simulink library "component_lib"  (R2023a)
settings: Solver=VariableStepAuto  StartTime=0.0  StopTime=10.0  RelTol=1e-3
undefined symbols (not defined in the file or in its folder): ECCV_r, par, R1234yf_ph, V_nom
libraries: base_lib x258, $bdroot x212, simulink x2, slpidlib x1
(part 4 of 7)

== system component_lib/Fuel Cell System/Subsystem1 ==
  note: Rolling Fuel Consumption Calculation [kg/100km]
  In1 : Inport
  Add1 : Sum
  Constant6 : Constant
  Constant7 : Constant  Value=100e3
  Demux : Demux
  Divide : Product  Inputs=**/
  Gain1 : Gain  Gain=-1
  Integrator : Integrator
  SC0002_signalRead11 : $bdroot/Data & Control/SC0002_signalRead  SigName=fuelConsumption
  SC0002_signalRead5 : $bdroot/Data & Control/SC0002_signalRead  SigName=hydrogenFlow
  SC0003_signalWrite1 : $bdroot/Data & Control/SC0003_signalWrite  SigName=distance
  Terminator : Terminator
  Terminator1 : Terminator
  Terminator2 : Terminator
  wires:
  Integrator/1 -> Divide/1
  Constant7/1 -> Divide/2
  SC0003_signalWrite1/1 -> Add1/1
  Demux/1 -> Gain1/1
  Add1/1 -> Divide/3
  Constant6/1 -> Add1/2
  Divide/1 -> SC0002_signalRead11/1
  Gain1/1 -> SC0002_signalRead5/1, Integrator/1
  In1/1 -> Demux/1
  Demux/3 -> Terminator1/1
  Demux/4 -> Terminator2/1
  Demux/2 -> Terminator/1

== system component_lib/Gas Exchange/GE0001_humidGasSupply ==
  Constant : Constant  Value=par.p_tot
  Constant1 : Constant  Value=par.RH
  Constant2 : Constant  Value=par.T
  Constant3 : Constant  Value=par.x_H2
  Constant4 : Constant  Value=par.x_O2
  F0010_pressureSupply.m : base_lib/F0010_gasFlow/F0010_pressureSupply.m  SystemSampleTime=-1  VariantActivationTime=update diagram  Latency=0  AutoFrameSizeCalculation=off
  F0010_vaporSaturationPressure.m : base_lib/F0010_gasFlow/F0010_vaporSaturationPressure.m  SystemSampleTime=-1  VariantActivationTime=update diagram  Latency=0  AutoFrameSizeCalculation=off
  p (p x 4) : Outport
  T [K] : Outport  Port=2
  wires:
  Constant2/1 -> T [K]/1, F0010_vaporSaturationPressure.m/1
  Constant/1 -> F0010_pressureSupply.m/1
  F0010_vaporSaturationPressure.m/1 -> F0010_pressureSupply.m/5
  Constant1/1 -> F0010_pressureSupply.m/4
  Constant3/1 -> F0010_pressureSupply.m/2
  Constant4/1 -> F0010_pressureSupply.m/3
  F0010_pressureSupply.m/1 -> p (p x 4)/1

== system component_lib/Gas Exchange/GE0002_dynHumidGasSupply ==
  T [K] : Inport
  p_ref [Pa] : Inport  Port=2
  RH [-] : Inport  Port=3
  Constant : Constant  Value=x_H2_dry
  Constant1 : Constant  Value=x_O2_dry
  F0010_pressureSupply.m : base_lib/F0010_gasFlow/F0010_pressureSupply.m  SystemSampleTime=-1  VariantActivationTime=update diagram  Latency=0  AutoFrameSizeCalculation=off
  F0010_vaporSaturationPressure.m : base_lib/F0010_gasFlow/F0010_vaporSaturationPressure.m  SystemSampleTime=-1  VariantActivationTime=update diagram  Latency=0  AutoFrameSizeCalculation=off
  p (p x 4) : Outport
  T_out [K] : Outport  Port=2
  wires:
  p_ref [Pa]/1 -> F0010_pressureSupply.m/1
  T [K]/1 -> F0010_vaporSaturationPressure.m/1, T_out [K]/1
  F0010_vaporSaturationPressure.m/1 -> F0010_pressureSupply.m/5
  RH [-]/1 -> F0010_pressureSupply.m/4
  F0010_pressureSupply.m/1 -> p (p x 4)/1
  Constant/1 -> F0010_pressureSupply.m/2
  Constant1/1 -> F0010_pressureSupply.m/3

== system component_lib/Gas Exchange/GE0007_hydrogenTank ==
  W_H2 [kg/s] : Inport
  Actuator dynamics : TransferFcn  Denominator=[0.1 1]
  Constant : Constant  Value=0
  Constant2 : Constant  Value=par.V
  Constant3 : Constant  Value=par.T_tank
  Constant4 : Constant  Value=0
  Constant5 : Constant  Value=par.m0
  Constant6 : Constant  Value=par.m0
  Constant7 : Constant  Value=par.M_j(1)
  Constant8 : Constant  Value=par.init_SOC
  Constant9 : Constant  Value=0
  Divide{,1..2,4} (4 alike) : Product  Inputs=*/
  F0005_enthalpy.m : base_lib/F0005_h2Thermodynamics/F0005_enthalpy.m  SystemSampleTime=-1  VariantActivationTime=update diagram  Latency=0  AutoFrameSizeCalculation=off
  F0005_pressure.m : base_lib/F0005_h2Thermodynamics/F0005_pressure.m  SystemSampleTime=-1  VariantActivationTime=update diagram  Latency=0  AutoFrameSizeCalculation=off
  Gain : Gain  Gain=-1
  Hydrogen ideal gas molar specific heat : Constant  Value=par.cp_j(1) .* par.M_j(1);
  Integrator Limited : Integrator  InitialConditionSource=external  LimitOutput=on  LowerSaturationLimit=0
  Mux : Mux
  Product : Product
  Standard state molar enthalpy : Constant  Value=par.h0
  Sum : Sum  Inputs=|+-
  Sum1 : Sum  Inputs=|++
  standard state temperature : Constant  Value=par.T0
  W [kg/s] : Outport
  T [K] : Outport  Port=2
  SOC [-] : Outport  Port=3
  p _tank [Pa] : Outport  Port=4
  wires:
  Integrator Limited/1 -> Divide1/1, Divide2/1
  Constant2/1 -> Divide1/2
  Constant3/1 -> F0005_pressure.m/1, F0005_enthalpy.m/1
  F0005_pressure.m/1 -> p _tank [Pa]/1
  Divide2/1 -> SOC [-]/1
  Hydrogen ideal gas molar specific heat/1 -> Divide/2
  Divide1/1 -> Divide4/1
  Constant7/1 -> Divide4/2
  Divide4/1 -> F0005_enthalpy.m/2, F0005_pressure.m/2
  F0005_enthalpy.m/1 -> Sum/1
  Standard state molar enthalpy/1 -> Sum/2
  Sum/1 -> Divide/1
  Divide/1 -> Sum1/1
  standard state temperature/1 -> Sum1/2
  Sum1/1 -> T [K]/1
  Constant5/1 -> Divide2/2
  Constant6/1 -> Product/1
  Product/1 -> Integrator Limited/2
  Constant8/1 -> Product/2
  Constant9/1 -> Mux/4
  Constant/1 -> Mux/2
  Constant4/1 -> Mux/3
  Actuator dynamics/1 -> Gain/1, Mux/1
  Mux/1 -> W [kg/s]/1
  Gain/1 -> Integrator Limited/1
  W_H2 [kg/s]/1 -> Actuator dynamics/1

== system component_lib/Gas Exchange/GE0008_gasProperties ==
  p (p x 4) : Inport
  T [K] : Inport  Port=2
  Demux : Demux
  Divide : Product  Inputs=*/
  F0010_vaporSaturationPressure.m : base_lib/F0010_gasFlow/F0010_vaporSaturationPressure.m  SystemSampleTime=-1  VariantActivationTime=update diagram  Latency=0  AutoFrameSizeCalculation=off
  Mux : Mux
  Sum : Sum  Inputs=|+|
  p [Pa] : Outport
  RH [-] : Outport  Port=2
  wires:
  Sum/1 -> p [Pa]/1
  p (p x 4)/1 -> Demux/1
  Demux/1 -> Mux/1
  Demux/2 -> Mux/2
  Demux/3 -> Divide/1, Mux/3
  Demux/4 -> Mux/4
  Mux/1 -> Sum/1
  Divide/1 -> RH [-]/1
  F0010_vaporSaturationPressure.m/1 -> Divide/2
  T [K]/1 -> F0010_vaporSaturationPressure.m/1

== system component_lib/Gas Exchange/GE0009_controlVolume ==
  note: Pressure
  note: Mass flow contribution
      | to pressure dynamics
  dW [kg/s x 4] : Inport
  T [K] : Inport  Port=2
  Constant : Constant  Value=par.p0
  Constant1 : Constant  Value=par.RH0
  Constant3 : Constant  Value=par.V
  Constant5 : Constant  Value=par.x0_H2
  Constant6 : Constant  Value=par.x0_O2
  Divide1 : Product  Inputs=***/
  F0010_pressureSupply.m : base_lib/F0010_gasFlow/F0010_pressureSupply.m  SystemSampleTime=-1  VariantActivationTime=update diagram  Latency=0  AutoFrameSizeCalculation=off
      settings: LibrarySourceBlock=|
      | simulink/User-Defined
      | Functions/MATLAB Function
  F0010_vaporSaturationPressure.m : base_lib/F0010_gasFlow/F0010_vaporSaturationPressure.m  SystemSampleTime=-1  VariantActivationTime=update diagram  Latency=0  AutoFrameSizeCalculation=off
      settings: LibrarySourceBlock=|
      | simulink/User-Defined
      | Functions/MATLAB Function
  Gas constants : Constant  Value=par.R_j
  Integrator Limited1 : Integrator  InitialConditionSource=external  LimitOutput=on  LowerSaturationLimit=0
  p [Pa x 4] : Outport
  wires:
  Integrator Limited1/1 -> p [Pa x 4]/1
  Constant/1 -> F0010_pressureSupply.m/1
  F0010_pressureSupply.m/1 -> Integrator Limited1/2
  dW [kg/s x 4]/1 -> Divide1/1
  Divide1/1 -> Integrator Limited1/1
  Constant3/1 -> Divide1/4
  Gas constants/1 -> Divide1/2
  F0010_vaporSaturationPressure.m/1 -> F0010_pressureSupply.m/5
  Constant1/1 -> F0010_pressureSupply.m/4
  Constant5/1 -> F0010_pressureSupply.m/2
  Constant6/1 -> F0010_pressureSupply.m/3
  T [K]/1 -> F0010_vaporSaturationPressure.m/1, Divide1/3

== system component_lib/Gas Exchange/GE0010_compressibleRestriction ==
  p_us [Pa x 4] : Inport
  T_us [K] : Inport  Port=2
  p_ds [Pa x 4] : Inport  Port=3
  Area : Constant  Value=pi*(D_t/2)^2
  F0010_compressibleRestriction.m : base_lib/F0010_gasFlow/F0010_compressibleRestriction.m  SystemSampleTime=-1  VariantActivationTime=update diagram  Latency=0  AutoFrameSizeCalculation=off
      settings: LibrarySourceBlock=|
      | simulink/User-Defined
      | Functions/MATLAB Function
  F0010_mixtureProperties.m : base_lib/F0010_gasFlow/F0010_mixtureProperties.m  SystemSampleTime=-1  VariantActivationTime=update diagram  Latency=0  AutoFrameSizeCalculation=off
      settings: LibrarySourceBlock=|
      | simulink/User-Defined
      | Functions/MATLAB Function
  F0010_multicomponentFlow.m : base_lib/F0010_gasFlow/F0010_multicomponentFlow.m  SystemSampleTime=-1  VariantActivationTime=update diagram  Latency=0  AutoFrameSizeCalculation=off
      settings: LibrarySourceBlock=|
      | simulink/User-Defined
      | Functions/MATLAB Function
  Sum : Sum  Inputs=+
  Sum1 : Sum  Inputs=+
  Terminator : Terminator
  Terminator1 : Terminator
  W [kg/s x 4] : Outport
  T_ds [K] : Outport  Port=2
  wires:
  T_us [K]/1 -> F0010_compressibleRestriction.m/3, T_ds [K]/1
  p_us [Pa x 4]/1 -> Sum/1, F0010_mixtureProperties.m/1, F0010_multicomponentFlow.m/1
  p_ds [Pa x 4]/1 -> Sum1/1
  Sum/1 -> F0010_compressibleRestriction.m/1
  Sum1/1 -> F0010_compressibleRestriction.m/2
  F0010_compressibleRestriction.m/1 -> F0010_multicomponentFlow.m/2
  F0010_multicomponentFlow.m/1 -> W [kg/s x 4]/1
  F0010_mixtureProperties.m/2 -> F0010_compressibleRestriction.m/4
  F0010_mixtureProperties.m/4 -> F0010_compressibleRestriction.m/5
  F0010_mixtureProperties.m/1 -> Terminator/1
  F0010_mixtureProperties.m/3 -> Terminator1/1
  Area/1 -> F0010_compressibleRestriction.m/6

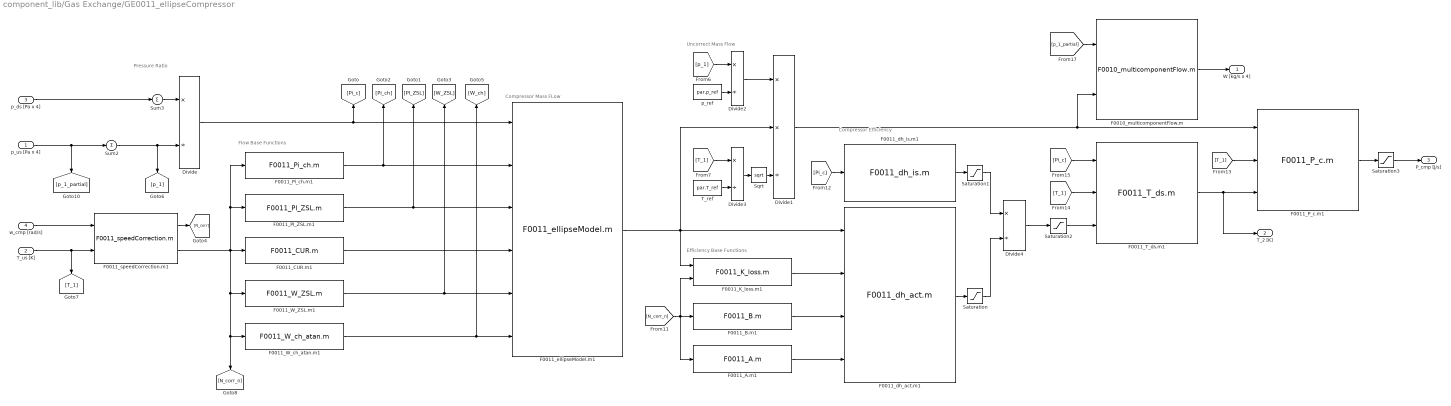
== system component_lib/Gas Exchange/GE0011_ellipseCompressor ==
  note: Compressor Mass FLow
  note: Compressor Efficiency
  note: Efficiency Base Functions
  note: Pressure Ratio
  note: Flow Base Functions
  note: Uncorrect Mass Flow
  p_us [Pa x 4] : Inport
  T_us [K] : Inport  Port=2
  p_ds [Pa x 4] : Inport  Port=3
  w_cmp [rad/s] : Inport  Port=4
  Divide{,2..4} (4 alike) : Product  Inputs=*/
  Divide1 : Product  Inputs=**/
  F0010_multicomponentFlow.m : base_lib/F0010_gasFlow/F0010_multicomponentFlow.m  SystemSampleTime=-1  VariantActivationTime=update diagram  Latency=0  AutoFrameSizeCalculation=off
      settings: LibrarySourceBlock=|
      | simulink/User-Defined
      | Functions/MATLAB Function
  F0011_A.m1 : base_lib/F0011_ellipseCompressor/F0011_A.m  SystemSampleTime=-1  VariantActivationTime=update diagram  Latency=0  AutoFrameSizeCalculation=off
      settings: LibrarySourceBlock=|
      | simulink/User-Defined
      | Functions/MATLAB Function
  F0011_B.m1 : base_lib/F0011_ellipseCompressor/F0011_B.m  SystemSampleTime=-1  VariantActivationTime=update diagram  Latency=0  AutoFrameSizeCalculation=off
      settings: LibrarySourceBlock=|
      | simulink/User-Defined
      | Functions/MATLAB Function
  F0011_CUR.m1 : base_lib/F0011_ellipseCompressor/F0011_CUR.m  SystemSampleTime=-1  VariantActivationTime=update diagram  Latency=0  AutoFrameSizeCalculation=off
      settings: LibrarySourceBlock=|
      | simulink/User-Defined
      | Functions/MATLAB Function
  F0011_K_loss.m1 : base_lib/F0011_ellipseCompressor/F0011_K_loss.m  SystemSampleTime=-1  VariantActivationTime=update diagram  Latency=0  AutoFrameSizeCalculation=off
      settings: LibrarySourceBlock=|
      | simulink/User-Defined
      | Functions/MATLAB Function
  F0011_PI_ZSL.m1 : base_lib/F0011_ellipseCompressor/F0011_PI_ZSL.m  SystemSampleTime=-1  VariantActivationTime=update diagram  Latency=0  AutoFrameSizeCalculation=off
      settings: LibrarySourceBlock=|
      | simulink/User-Defined
      | Functions/MATLAB Function
  F0011_P_c.m1 : base_lib/F0011_ellipseCompressor/F0011_P_c.m  SystemSampleTime=-1  VariantActivationTime=update diagram  Latency=0  AutoFrameSizeCalculation=off
      settings: LibrarySourceBlock=|
      | simulink/User-Defined
      | Functions/MATLAB Function
  F0011_Pi_ch.m1 : base_lib/F0011_ellipseCompressor/F0011_Pi_ch.m  SystemSampleTime=-1  VariantActivationTime=update diagram  Latency=0  AutoFrameSizeCalculation=off
      settings: LibrarySourceBlock=|
      | simulink/User-Defined
      | Functions/MATLAB Function
  F0011_T_ds.m1 : base_lib/F0011_ellipseCompressor/F0011_T_ds.m  SystemSampleTime=-1  VariantActivationTime=update diagram  Latency=0  AutoFrameSizeCalculation=off
      settings: LibrarySourceBlock=|
      | simulink/User-Defined
      | Functions/MATLAB Function
  F0011_W_ZSL.m1 : base_lib/F0011_ellipseCompressor/F0011_W_ZSL.m  SystemSampleTime=-1  VariantActivationTime=update diagram  Latency=0  AutoFrameSizeCalculation=off
      settings: LibrarySourceBlock=|
      | simulink/User-Defined
      | Functions/MATLAB Function
  F0011_W_ch_atan.m1 : base_lib/F0011_ellipseCompressor/F0011_W_ch_atan.m  SystemSampleTime=-1  VariantActivationTime=update diagram  Latency=0  AutoFrameSizeCalculation=off
      settings: LibrarySourceBlock=|
      | simulink/User-Defined
      | Functions/MATLAB Function
  F0011_dh_act.m1 : base_lib/F0011_ellipseCompressor/F0011_dh_act.m  SystemSampleTime=-1  VariantActivationTime=update diagram  Latency=0  AutoFrameSizeCalculation=off
      settings: LibrarySourceBlock=|
      | simulink/User-Defined
      | Functions/MATLAB Function
  F0011_dh_is.m1 : base_lib/F0011_ellipseCompressor/F0011_dh_is.m  SystemSampleTime=-1  VariantActivationTime=update diagram  Latency=0  AutoFrameSizeCalculation=off
      settings: LibrarySourceBlock=|
      | simulink/User-Defined
      | Functions/MATLAB Function
  F0011_ellipseModel.m1 : base_lib/F0011_ellipseCompressor/F0011_ellipseModel.m  SystemSampleTime=-1  VariantActivationTime=update diagram  Latency=0  AutoFrameSizeCalculation=off
      settings: LibrarySourceBlock=|
      | simulink/User-Defined
      | Functions/MATLAB Function
  F0011_speedCorrection.m1 : base_lib/F0011_ellipseCompressor/F0011_speedCorrection.m  SystemSampleTime=-1  VariantActivationTime=update diagram  Latency=0  AutoFrameSizeCalculation=off
      settings: LibrarySourceBlock=|
      | simulink/User-Defined
      | Functions/MATLAB Function
  Saturation : Saturate  UpperLimit=inf  LowerLimit=1e-4
  Saturation1 : Saturate  UpperLimit=inf  LowerLimit=1e-4
  Saturation2 : Saturate  UpperLimit=1  LowerLimit=1e-3
  Saturation3 : Saturate  UpperLimit=inf  LowerLimit=0
  Sqrt : Sqrt
  Sum2 : Sum  Inputs=|+|
  Sum3 : Sum  Inputs=|+|
  T_ref : Constant  Value=par.T_ref
  p_ref : Constant  Value=par.p_ref
  W [kg/s x 4] : Outport
  T_2 [K] : Outport  Port=2
  P_cmp [J/s] : Outport  Port=3
  wires:
  Sum3/1 -> Divide/1
  T_us [K]/1 -> F0011_speedCorrection.m1/2, [T_1]
  F0011_CUR.m1/1 -> F0011_ellipseModel.m1/4
  F0011_PI_ZSL.m1/1 -> F0011_ellipseModel.m1/3, [PI_ZSL]
  F0011_W_ZSL.m1/1 -> F0011_ellipseModel.m1/5, [W_ZSL]
  F0011_W_ch_atan.m1/1 -> F0011_ellipseModel.m1/6, [W_ch]
  F0011_speedCorrection.m1/2 -> F0011_CUR.m1/1, F0011_W_ZSL.m1/1, F0011_W_ch_atan.m1/1, [N_corr_n], F0011_PI_ZSL.m1/1, F0011_Pi_ch.m1/1
  Divide/1 -> F0011_ellipseModel.m1/1, [Pi_c]
  F0011_speedCorrection.m1/1 -> [N_corr]
  Divide1/1 -> F0011_P_c.m1/1, F0010_multicomponentFlow.m/2
  p_ref/1 -> Divide2/2
  Divide2/1 -> Divide1/1
  [p_1] -> Divide2/1
  [T_1] -> Divide3/1
  T_ref/1 -> Divide3/2
  Divide3/1 -> Sqrt/1
  Sqrt/1 -> Divide1/3
  F0011_Pi_ch.m1/1 -> F0011_ellipseModel.m1/2, [Pi_ch]
  F0011_K_loss.m1/1 -> F0011_dh_act.m1/2
  F0011_B.m1/1 -> F0011_dh_act.m1/3
  F0011_A.m1/1 -> F0011_dh_act.m1/4
  [N_corr_n] -> F0011_A.m1/1, F0011_B.m1/1, F0011_K_loss.m1/2
  [Pi_c] -> F0011_dh_is.m1/1
  F0011_dh_act.m1/1 -> Saturation/1
  F0011_dh_is.m1/1 -> Saturation1/1
  Saturation1/1 -> Divide4/1
  Saturation/1 -> Divide4/2
  Divide4/1 -> Saturation2/1
  Saturation2/1 -> F0011_T_ds.m1/3
  F0011_T_ds.m1/1 -> F0011_P_c.m1/3, T_2 [K]/1
  [T_1] -> F0011_P_c.m1/2
  [T_1] -> F0011_T_ds.m1/2
  [Pi_c] -> F0011_T_ds.m1/1
  w_cmp [rad/s]/1 -> F0011_speedCorrection.m1/1
  p_us [Pa x 4]/1 -> Sum2/1, [p_1_partial]
  Sum2/1 -> Divide/2, [p_1]
  [p_1_partial] -> F0010_multicomponentFlow.m/1
  F0010_multicomponentFlow.m/1 -> W [kg/s x 4]/1
  F0011_ellipseModel.m1/1 -> F0011_dh_act.m1/1, F0011_K_loss.m1/1, Divide1/2
  p_ds [Pa x 4]/1 -> Sum3/1
  F0011_P_c.m1/1 -> Saturation3/1
  Saturation3/1 -> P_cmp [J/s]/1

== system component_lib/Gas Exchange/GE0012_throttle ==
  p_us [Pa x 4] : Inport
  T_us [K] : Inport  Port=2
  p_ds [Pa x 4] : Inport  Port=3
  alpha [-] : Inport  Port=4
  F0010_compressibleRestriction.m : base_lib/F0010_gasFlow/F0010_compressibleRestriction.m  SystemSampleTime=-1  VariantActivationTime=update diagram  Latency=0  AutoFrameSizeCalculation=off
      settings: LibrarySourceBlock=|
      | simulink/User-Defined
      | Functions/MATLAB Function
  F0010_mixtureProperties.m : base_lib/F0010_gasFlow/F0010_mixtureProperties.m  SystemSampleTime=-1  VariantActivationTime=update diagram  Latency=0  AutoFrameSizeCalculation=off
      settings: LibrarySourceBlock=|
      | simulink/User-Defined
      | Functions/MATLAB Function
  F0010_multicomponentFlow.m : base_lib/F0010_gasFlow/F0010_multicomponentFlow.m  SystemSampleTime=-1  VariantActivationTime=update diagram  Latency=0  AutoFrameSizeCalculation=off
      settings: LibrarySourceBlock=|
      | simulink/User-Defined
      | Functions/MATLAB Function
  F0010_throttleArea.m : base_lib/F0010_gasFlow/F0010_throttleArea.m  SystemSampleTime=-1  VariantActivationTime=update diagram  Latency=0  AutoFrameSizeCalculation=off
      settings: LibrarySourceBlock=|
      | simulink/User-Defined
      | Functions/MATLAB Function
  Sum : Sum  Inputs=+
  Sum1 : Sum  Inputs=+
  Terminator : Terminator
  Terminator1 : Terminator
  W [kg/s x 4] : Outport
  T_out [K] : Outport  Port=2
  wires:
  T_us [K]/1 -> F0010_compressibleRestriction.m/3, T_out [K]/1
  p_us [Pa x 4]/1 -> Sum/1, F0010_mixtureProperties.m/1, F0010_multicomponentFlow.m/1
  p_ds [Pa x 4]/1 -> Sum1/1
  Sum/1 -> F0010_compressibleRestriction.m/1
  Sum1/1 -> F0010_compressibleRestriction.m/2
  F0010_compressibleRestriction.m/1 -> F0010_multicomponentFlow.m/2
  F0010_multicomponentFlow.m/1 -> W [kg/s x 4]/1
  F0010_mixtureProperties.m/2 -> F0010_compressibleRestriction.m/4
  F0010_mixtureProperties.m/4 -> F0010_compressibleRestriction.m/5
  F0010_mixtureProperties.m/1 -> Terminator/1
  F0010_mixtureProperties.m/3 -> Terminator1/1
  F0010_throttleArea.m/1 -> F0010_compressibleRestriction.m/6
  alpha [-]/1 -> F0010_throttleArea.m/1

== system component_lib/Gas Exchange/GE0013_ejector ==
  p_p [Pa x 4] : Inport
  T_p [K] : Inport  Port=2
  p_s [Pa x 4] : Inport  Port=3
  T_s [K] : Inport  Port=4
  p_b [Pa x 4] : Inport  Port=5
  Divide : Product  Inputs=*/
  F0010_ejectorModel.m : base_lib/F0010_gasFlow/F0010_ejectorModel.m  SystemSampleTime=-1  VariantActivationTime=update diagram  Latency=0  AutoFrameSizeCalculation=off
      settings: LibrarySourceBlock=|
      | simulink/User-Defined
      | Functions/MATLAB Function
  F0010_multicomponentFlow.m : base_lib/F0010_gasFlow/F0010_multicomponentFlow.m  SystemSampleTime=-1  VariantActivationTime=update diagram  Latency=0  AutoFrameSizeCalculation=off
  F0010_multicomponentFlow.m1 : base_lib/F0010_gasFlow/F0010_multicomponentFlow.m  SystemSampleTime=-1  VariantActivationTime=update diagram  Latency=0  AutoFrameSizeCalculation=off
  F0010_vaporSaturationPressure.m : base_lib/F0010_gasFlow/F0010_vaporSaturationPressure.m  SystemSampleTime=-1  VariantActivationTime=update diagram  Latency=0  AutoFrameSizeCalculation=off
  Selector : Selector  InputPortWidth=4  IndexOptions=Index vector (dialog)  Indices=3  OutputSizes=1
  Sum : Sum  Inputs=+
  Sum1 : Sum  Inputs=+
  Sum2 : Sum  Inputs=+
  W_p [kg/s] : Outport
  W_s [kg/s] : Outport  Port=2
  phi [-] : Outport  Port=3
  w [-] : Outport  Port=4
  wires:
  p_p [Pa x 4]/1 -> Sum/1, [P_p]
  Sum/1 -> F0010_ejectorModel.m/1
  p_s [Pa x 4]/1 -> Sum1/1, [P_s]
  Sum1/1 -> F0010_ejectorModel.m/2
  Sum2/1 -> F0010_ejectorModel.m/3
  p_b [Pa x 4]/1 -> Sum2/1
  F0010_ejectorModel.m/1 -> F0010_multicomponentFlow.m/2
  F0010_multicomponentFlow.m/1 -> W_p [kg/s]/1
  F0010_ejectorModel.m/2 -> F0010_multicomponentFlow.m1/2
  F0010_multicomponentFlow.m1/1 -> W_s [kg/s]/1
  [P_p] -> F0010_multicomponentFlow.m/1
  [P_s] -> F0010_multicomponentFlow.m1/1
  F0010_ejectorModel.m/3 -> phi [-]/1
  T_p [K]/1 -> F0010_ejectorModel.m/4, [T_p]
  T_s [K]/1 -> F0010_vaporSaturationPressure.m/1
  [P_s] -> Selector/1
  Divide/1 -> F0010_ejectorModel.m/6
  Selector/1 -> Divide/1
  F0010_vaporSaturationPressure.m/1 -> F0010_ejectorModel.m/5, Divide/2
  F0010_ejectorModel.m/4 -> w [-]/1

== system component_lib/Gas Exchange/GE0014_flowValve ==
  p_us [Pa x 4] : Inport
  T_us [K] : Inport  Port=2
  p_ds [Pa x 4] : Inport  Port=3
  open [-] : Inport  Port=4
  Area : Constant  Value=pi*(D_t/2)^2
  F0010_compressibleRestriction.m : base_lib/F0010_gasFlow/F0010_compressibleRestriction.m  SystemSampleTime=-1  VariantActivationTime=update diagram  Latency=0  AutoFrameSizeCalculation=off
      settings: LibrarySourceBlock=|
      | simulink/User-Defined
      | Functions/MATLAB Function
  F0010_mixtureProperties.m : base_lib/F0010_gasFlow/F0010_mixtureProperties.m  SystemSampleTime=-1  VariantActivationTime=update diagram  Latency=0  AutoFrameSizeCalculation=off
      settings: LibrarySourceBlock=|
      | simulink/User-Defined
      | Functions/MATLAB Function
  F0010_multicomponentFlow.m : base_lib/F0010_gasFlow/F0010_multicomponentFlow.m  SystemSampleTime=-1  VariantActivationTime=update diagram  Latency=0  AutoFrameSizeCalculation=off
      settings: LibrarySourceBlock=|
      | simulink/User-Defined
      | Functions/MATLAB Function
  Product : Product
  Sum : Sum  Inputs=+
  Sum1 : Sum  Inputs=+
  Terminator : Terminator
  Terminator1 : Terminator
  W [kg/s x 4] : Outport
  T_ds [K] : Outport  Port=2
  wires:
  T_us [K]/1 -> F0010_compressibleRestriction.m/3, T_ds [K]/1
  p_us [Pa x 4]/1 -> Sum/1, F0010_mixtureProperties.m/1, F0010_multicomponentFlow.m/1
  p_ds [Pa x 4]/1 -> Sum1/1
  Sum/1 -> F0010_compressibleRestriction.m/1
  Sum1/1 -> F0010_compressibleRestriction.m/2
  F0010_compressibleRestriction.m/1 -> F0010_multicomponentFlow.m/2
  F0010_multicomponentFlow.m/1 -> W [kg/s x 4]/1
  F0010_mixtureProperties.m/2 -> F0010_compressibleRestriction.m/4
  F0010_mixtureProperties.m/4 -> F0010_compressibleRestriction.m/5
  F0010_mixtureProperties.m/1 -> Terminator/1
  F0010_mixtureProperties.m/3 -> Terminator1/1
  Area/1 -> Product/1
  Product/1 -> F0010_compressibleRestriction.m/6
  open [-]/1 -> Product/2

== system component_lib/Gas Exchange/GE0015_linearRestriction ==
  p_us [Pa x 4] : Inport
  p_ds [Pa x 4] : Inport  Port=2
  F0010_linearRestriction.m : base_lib/F0010_gasFlow/F0010_linearRestriction.m  SystemSampleTime=-1  VariantActivationTime=update diagram  Latency=0  AutoFrameSizeCalculation=off
      settings: LibrarySourceBlock=|
      | simulink/User-Defined
      | Functions/MATLAB Function
  F0010_multicomponentFlow.m : base_lib/F0010_gasFlow/F0010_multicomponentFlow.m  SystemSampleTime=-1  VariantActivationTime=update diagram  Latency=0  AutoFrameSizeCalculation=off
      settings: LibrarySourceBlock=|
      | simulink/User-Defined
      | Functions/MATLAB Function
  Sum : Sum  Inputs=+
  Sum1 : Sum  Inputs=+
  W [kg/s x 4] : Outport
  wires:
  F0010_multicomponentFlow.m/1 -> W [kg/s x 4]/1
  p_us [Pa x 4]/1 -> F0010_multicomponentFlow.m/1, Sum/1
  p_ds [Pa x 4]/1 -> Sum1/1
  Sum/1 -> F0010_linearRestriction.m/1
  Sum1/1 -> F0010_linearRestriction.m/2
  F0010_linearRestriction.m/1 -> F0010_multicomponentFlow.m/2

== system component_lib/Gas Exchange/GE0016_simpleCompressor ==
  W [kg/s] : Inport
  p2 [Pa] : Inport  Port=2
  T1 [K] : Inport  Port=3
  p1 [Pa] : Inport  Port=4
  Constant : Constant  Value=eta
  F0007_compressorPower.m : base_lib/F0019_simpleCompressor/F0007_compressorPower.m  SystemSampleTime=-1  VariantActivationTime=update diagram  Latency=0  AutoFrameSizeCalculation=off
  F0007_compressorTemperature.m : base_lib/F0019_simpleCompressor/F0007_compressorTemperature.m  SystemSampleTime=-1  VariantActivationTime=update diagram  Latency=0  AutoFrameSizeCalculation=off
  P_cmp [J/s] : Outport
  wires:
  T1 [K]/1 -> F0007_compressorTemperature.m/3, F0007_compressorPower.m/2
  F0007_compressorTemperature.m/1 -> F0007_compressorPower.m/3
  W [kg/s]/1 -> F0007_compressorPower.m/1
  F0007_compressorPower.m/1 -> P_cmp [J/s]/1
  Constant/1 -> F0007_compressorTemperature.m/4
  p2 [Pa]/1 -> F0007_compressorTemperature.m/2
  p1 [Pa]/1 -> F0007_compressorTemperature.m/1

== system component_lib/Gas Exchange/GE0017_humidifier ==
  p [Pa x 4]) : Inport
  RH_ref [-] : Inport  Port=2
  T [K] : Inport  Port=3
  Demux : Demux
  F0003_vaporActivity.m : base_lib/F0003_pukrushpan2004/F0003_vaporActivity.m  SystemSampleTime=-1  VariantActivationTime=update diagram  Latency=0  AutoFrameSizeCalculation=off
  F0010_vaporSaturationPressure.m : base_lib/F0010_gasFlow/F0010_vaporSaturationPressure.m  SystemSampleTime=-1  VariantActivationTime=update diagram  Latency=0  AutoFrameSizeCalculation=off
      settings: LibrarySourceBlock=|
      | simulink/User-Defined
      | Functions/MATLAB Function
  Gain : Gain  Gain=gain
  Mux : Mux
  Sum : Sum  Inputs=|+-
  W [kg/s x 4] : Outport
  wires:
  Sum/1 -> Gain/1
  F0010_vaporSaturationPressure.m/1 -> F0003_vaporActivity.m/2
  Demux/3 -> F0003_vaporActivity.m/1
  Gain/1 -> Mux/3
  p [Pa x 4])/1 -> Demux/1
  T [K]/1 -> F0010_vaporSaturationPressure.m/1
  Mux/1 -> W [kg/s x 4]/1
  F0003_vaporActivity.m/1 -> Sum/2
  RH_ref [-]/1 -> Sum/1

== system component_lib/Gas Exchange/GE0018_condenser ==
  p_in [Pa x 4]) : Inport
  T_cds [K] : Inport  Port=2
  Constant : Constant
  Demux : Demux
  F0003_vaporActivity.m : base_lib/F0003_pukrushpan2004/F0003_vaporActivity.m  SystemSampleTime=-1  VariantActivationTime=update diagram  Latency=0  AutoFrameSizeCalculation=off
  F0010_vaporSaturationPressure.m : base_lib/F0010_gasFlow/F0010_vaporSaturationPressure.m  SystemSampleTime=-1  VariantActivationTime=update diagram  Latency=0  AutoFrameSizeCalculation=off
      settings: LibrarySourceBlock=|
      | simulink/User-Defined
      | Functions/MATLAB Function
  Gain : Gain  Gain=gain
  Mux : Mux
  Saturation : Saturate  UpperLimit=inf  LowerLimit=0  ZeroCross=off
  Sum : Sum  Inputs=|+-
  W [kg/s x 4] : Outport
  wires:
  Demux/3 -> F0003_vaporActivity.m/1
  p_in [Pa x 4])/1 -> Demux/1
  F0010_vaporSaturationPressure.m/1 -> F0003_vaporActivity.m/2
  T_cds [K]/1 -> F0010_vaporSaturationPressure.m/1
  Constant/1 -> Sum/2
  Mux/1 -> W [kg/s x 4]/1
  Saturation/1 -> Gain/1
  Sum/1 -> Saturation/1
  Gain/1 -> Mux/3
  F0003_vaporActivity.m/1 -> Sum/1

== system component_lib/Gas Exchange/GE0019_expander ==
  W [kg/s] : Inport
  p3 [Pa] : Inport  Port=2
  T3 [K] : Inport  Port=3
  p4 [Pa] : Inport  Port=4
  N [rpm] : Inport  Port=5
  F0026_turbine.m : base_lib/F0026_turbine/F0026_turbine.m  SystemSampleTime=-1  VariantActivationTime=update diagram  Latency=0  AutoFrameSizeCalculation=off
      settings: LibrarySourceBlock=|
      | simulink/User-Defined
      | Functions/MATLAB Function
  Saturation : Saturate  UpperLimit=200e3  LowerLimit=0
  P [J/s] : Outport
  eta [-] : Outport  Port=2
  T4 [K] : Outport  Port=3
  wires:
  N [rpm]/1 -> Saturation/1
  Saturation/1 -> F0026_turbine.m/5
  F0026_turbine.m/1 -> P [J/s]/1
  F0026_turbine.m/2 -> eta [-]/1
  F0026_turbine.m/3 -> T4 [K]/1
  W [kg/s]/1 -> F0026_turbine.m/1
  p3 [Pa]/1 -> F0026_turbine.m/2
  T3 [K]/1 -> F0026_turbine.m/4
  p4 [Pa]/1 -> F0026_turbine.m/3

== system component_lib/Gas Exchange/GE0020_compressor ==
  note: Compressor Efficiency
  note: Compressor Pressure Ratio
  note: Efficiency Base Functions
  note: Flow Base Functions
  W [kg/s] : Inport
  p1 [Pa] : Inport  Port=2
  T1 [K] : Inport  Port=3
  N [rpm] : Inport  Port=4
  Divide4 : Product  Inputs=*/
  F0011_A.m1 : base_lib/F0011_ellipseCompressor/F0011_A.m  SystemSampleTime=-1  VariantActivationTime=update diagram  Latency=0  AutoFrameSizeCalculation=off
      settings: LibrarySourceBlock=|
      | simulink/User-Defined
      | Functions/MATLAB Function
  F0011_B.m1 : base_lib/F0011_ellipseCompressor/F0011_B.m  SystemSampleTime=-1  VariantActivationTime=update diagram  Latency=0  AutoFrameSizeCalculation=off
      settings: LibrarySourceBlock=|
      | simulink/User-Defined
      | Functions/MATLAB Function
  F0011_CUR.m1 : base_lib/F0011_ellipseCompressor/F0011_CUR.m  SystemSampleTime=-1  VariantActivationTime=update diagram  Latency=0  AutoFrameSizeCalculation=off
      settings: LibrarySourceBlock=|
      | simulink/User-Defined
      | Functions/MATLAB Function
  F0011_K_loss.m1 : base_lib/F0011_ellipseCompressor/F0011_K_loss.m  SystemSampleTime=-1  VariantActivationTime=update diagram  Latency=0  AutoFrameSizeCalculation=off
      settings: LibrarySourceBlock=|
      | simulink/User-Defined
      | Functions/MATLAB Function
  F0011_PI_ZSL.m1 : base_lib/F0011_ellipseCompressor/F0011_PI_ZSL.m  SystemSampleTime=-1  VariantActivationTime=update diagram  Latency=0  AutoFrameSizeCalculation=off
      settings: LibrarySourceBlock=|
      | simulink/User-Defined
      | Functions/MATLAB Function
  F0011_P_c.m1 : base_lib/F0011_ellipseCompressor/F0011_P_c.m  SystemSampleTime=-1  VariantActivationTime=update diagram  Latency=0  AutoFrameSizeCalculation=off
      settings: LibrarySourceBlock=|
      | simulink/User-Defined
      | Functions/MATLAB Function
  F0011_Pi_ch.m1 : base_lib/F0011_ellipseCompressor/F0011_Pi_ch.m  SystemSampleTime=-1  VariantActivationTime=update diagram  Latency=0  AutoFrameSizeCalculation=off
      settings: LibrarySourceBlock=|
      | simulink/User-Defined
      | Functions/MATLAB Function
  F0011_T_ds.m1 : base_lib/F0011_ellipseCompressor/F0011_T_ds.m  SystemSampleTime=-1  VariantActivationTime=update diagram  Latency=0  AutoFrameSizeCalculation=off
      settings: LibrarySourceBlock=|
      | simulink/User-Defined
      | Functions/MATLAB Function
  F0011_W_ZSL.m1 : base_lib/F0011_ellipseCompressor/F0011_W_ZSL.m  SystemSampleTime=-1  VariantActivationTime=update diagram  Latency=0  AutoFrameSizeCalculation=off
      settings: LibrarySourceBlock=|
      | simulink/User-Defined
      | Functions/MATLAB Function
  F0011_W_ch_atan.m1 : base_lib/F0011_ellipseCompressor/F0011_W_ch_atan.m  SystemSampleTime=-1  VariantActivationTime=update diagram  Latency=0  AutoFrameSizeCalculation=off
      settings: LibrarySourceBlock=|
      | simulink/User-Defined
      | Functions/MATLAB Function
  F0011_dh_act.m1 : base_lib/F0011_ellipseCompressor/F0011_dh_act.m  SystemSampleTime=-1  VariantActivationTime=update diagram  Latency=0  AutoFrameSizeCalculation=off
      settings: LibrarySourceBlock=|
      | simulink/User-Defined
      | Functions/MATLAB Function
  F0011_dh_is.m1 : base_lib/F0011_ellipseCompressor/F0011_dh_is.m  SystemSampleTime=-1  VariantActivationTime=update diagram  Latency=0  AutoFrameSizeCalculation=off
      settings: LibrarySourceBlock=|
      | simulink/User-Defined
      | Functions/MATLAB Function
  F0011_ellipseModelPressure.m : base_lib/F0011_ellipseCompressor/F0011_ellipseModelPressure.m  SystemSampleTime=-1  VariantActivationTime=update diagram  Latency=0  AutoFrameSizeCalculation=off
      settings: LibrarySourceBlock=|
      | simulink/User-Defined
      | Functions/MATLAB Function
  F0011_flowCorrection.m : base_lib/F0011_ellipseCompressor/F0011_flowCorrection.m  SystemSampleTime=-1  VariantActivationTime=update diagram  Latency=0  AutoFrameSizeCalculation=off
      settings: LibrarySourceBlock=|
      | simulink/User-Defined
      | Functions/MATLAB Function
  F0011_speedCorrection.m1 : base_lib/F0011_ellipseCompressor/F0011_speedCorrection.m  SystemSampleTime=-1  VariantActivationTime=update diagram  Latency=0  AutoFrameSizeCalculation=off
      settings: LibrarySourceBlock=|
      | simulink/User-Defined
      | Functions/MATLAB Function
  Gain : Gain  Gain=pi / 30
  Product : Product
  Saturation : Saturate  UpperLimit=inf  LowerLimit=1e-4
  Saturation1 : Saturate  UpperLimit=inf  LowerLimit=1e-4
  Saturation2 : Saturate  UpperLimit=1  LowerLimit=1e-3
  Saturation3 : Saturate  UpperLimit=inf  LowerLimit=0
  Sum2 : Sum  Inputs=|+|
  P [J/s] : Outport
  p2 [Pa] : Outport  Port=2
  T2 [K] : Outport  Port=3
  wires:
  [T1] -> F0011_P_c.m1/2
  Saturation3/1 -> P [J/s]/1
  F0011_P_c.m1/1 -> Saturation3/1
  T1 [K]/1 -> F0011_flowCorrection.m/3, [T1], F0011_speedCorrection.m1/2
  F0011_W_ZSL.m1/1 -> F0011_ellipseModelPressure.m/5, [W_ZSL]
  p1 [Pa]/1 -> [p1], Sum2/1
  [Pi_c] -> F0011_T_ds.m1/1
  Saturation/1 -> Divide4/2
  [T1] -> F0011_T_ds.m1/2
  Saturation1/1 -> Divide4/1
  Divide4/1 -> Saturation2/1
  F0011_dh_is.m1/1 -> Saturation1/1
  F0011_speedCorrection.m1/2 -> F0011_CUR.m1/1, F0011_W_ZSL.m1/1, F0011_W_ch_atan.m1/1, [N_corr_n], F0011_PI_ZSL.m1/1, F0011_Pi_ch.m1/1
  F0011_B.m1/1 -> F0011_dh_act.m1/3
  F0011_Pi_ch.m1/1 -> F0011_ellipseModelPressure.m/2, [Pi_ch]
  F0011_T_ds.m1/1 -> T2 [K]/1, F0011_P_c.m1/3
  F0011_dh_act.m1/1 -> Saturation/1
  F0011_flowCorrection.m/1 -> F0011_ellipseModelPressure.m/1, [W_corr]
  Saturation2/1 -> F0011_T_ds.m1/3
  [Pi_c] -> F0011_dh_is.m1/1
  F0011_W_ch_atan.m1/1 -> F0011_ellipseModelPressure.m/6, [W_ch]
  [N_corr_n] -> F0011_A.m1/1, F0011_B.m1/1
  F0011_A.m1/1 -> F0011_dh_act.m1/4
  F0011_speedCorrection.m1/1 -> [N_corr]
  F0011_K_loss.m1/1 -> F0011_dh_act.m1/2
  F0011_PI_ZSL.m1/1 -> F0011_ellipseModelPressure.m/3, [PI_ZSL]
  F0011_CUR.m1/1 -> F0011_ellipseModelPressure.m/4
  Gain/1 -> F0011_speedCorrection.m1/1
  N [rpm]/1 -> Gain/1
  W [kg/s]/1 -> [W], F0011_flowCorrection.m/1
  Sum2/1 -> F0011_flowCorrection.m/2
  F0011_ellipseModelPressure.m/1 -> [Pi_c]
  [W_corr] -> F0011_K_loss.m1/1
  [N_corr] -> F0011_K_loss.m1/2
  [W] -> F0011_P_c.m1/1
  [Pi_c] -> Product/2
  [p1] -> Product/1
  Product/1 -> p2 [Pa]/1

== system component_lib/Mission/MN0001_profile ==
  v [m/s] : Inport
  Altitute lookup table : Lookup_n-D  NumberOfTableDimensions=1  BreakpointsForDimension1=ECCV_r.distance  Table=ECCV_r.altitude  InternalRulePriority=Speed  RndMeth=Simplest
  Compare To Constant : simulink/Logic and Bit Operations/Compare To Constant  relop=>=  const=ECCV_r.distance(end-N_lookahead)  OutDataTypeStr=boolean
  Constant1 : Constant  Value=ECCV_r.slope
  Find current index of distance vector : Lookup_n-D  NumberOfTableDimensions=1  BreakpointsForDimension1=ECCV_r.distance  Table=1:length(ECCV_r.distance)  InterpMethod=Nearest  InternalRulePriority=Speed  RndMeth=Simplest
  Initial position : Constant  Value=x0
  Integrator1 : Integrator  InitialConditionSource=external
  Selector : Selector  InputPortWidth=length(ECCV_r.slope)  IndexOptions=Starting index (port)  Indices=[1 3]  OutputSizes=N_lookahead
  Slope lookup table : Lookup_n-D  NumberOfTableDimensions=1  BreakpointsForDimension1=ECCV_r.distance  Table=ECCV_r.slope  InternalRulePriority=Speed  RndMeth=Simplest
  Stop Simulation : Stop
  slope [rad] : Outport
  altitude [m] : Outport  Port=2
  distance [m] : Outport  Port=3
  slope_lookahead [rad] : Outport  Port=4
  wires:
  Integrator1/1 -> Find current index of distance vector/1, Altitute lookup table/1, Slope lookup table/1, distance [m]/1, Compare To Constant/1
  Slope lookup table/1 -> slope [rad]/1
  Altitute lookup table/1 -> altitude [m]/1
  Compare To Constant/1 -> Stop Simulation/1
  Selector/1 -> slope_lookahead [rad]/1
  Constant1/1 -> Selector/1
  Find current index of distance vector/1 -> Selector/2
  Initial position/1 -> Integrator1/2
  v [m/s]/1 -> Integrator1/1

== system component_lib/Mission/MN0002_ambient ==
  note: 4 % per km decrease
  altitude [m] : Inport
  Constant : Constant  Value=RH_0
  F0018_troposphereModel.m : base_lib/F0018_ambientProperties/F0018_troposphereModel.m  SystemSampleTime=-1  VariantActivationTime=update diagram  Latency=0  AutoFrameSizeCalculation=off
  Gain : Gain  Gain=0.04e-3
  Product : Product
  Sum : Sum  Inputs=|+-
  T [K] : Outport
  p [Pa] : Outport  Port=2
  RH [-] : Outport  Port=3
  wires:
  F0018_troposphereModel.m/2 -> T [K]/1
  F0018_troposphereModel.m/1 -> p [Pa]/1
  altitude [m]/1 -> Gain/1, F0018_troposphereModel.m/1
  Gain/1 -> Product/2
  Constant/1 -> Sum/1, Product/1
  Product/1 -> Sum/2
  Sum/1 -> RH [-]/1

== system component_lib/Powertrain/PT0001_simpleVehicle ==
  note: Tractive force
  Tq_in [Nm] : Inport
  alpha [rad] : Inport  Port=2
  brake [-] : Inport  Port=3
  Abs : Abs  SaturateOnIntegerOverflow=off
  Abs1 : Abs  SaturateOnIntegerOverflow=off
  Constant : Constant  Value=par.r_w
  Divide : Product  Inputs=*/
  Divide1 : Product  Inputs=*/
  F0006_airDrag.m : base_lib/F0006_truckBenchmark/F0006_airDrag.m  SystemSampleTime=-1  VariantActivationTime=update diagram  Latency=0  AutoFrameSizeCalculation=off
  F0006_brakeForce.m : base_lib/F0006_truckBenchmark/F0006_brakeForce.m  SystemSampleTime=-1  VariantActivationTime=update diagram  Latency=0  AutoFrameSizeCalculation=off
  F0006_gravitationalForce.m : base_lib/F0006_truckBenchmark/F0006_gravitationalForce.m  SystemSampleTime=-1  VariantActivationTime=update diagram  Latency=0  AutoFrameSizeCalculation=off
  F0006_rollingResistance.m : base_lib/F0006_truckBenchmark/F0006_rollingResistance.m  SystemSampleTime=-1  VariantActivationTime=update diagram  Latency=0  AutoFrameSizeCalculation=off
  Gain : Gain  Gain=1/par.m
  Initial speed : Constant  Value=par.v0
  Integrator2 : Integrator  InitialConditionSource=external
  Sum : Sum  Inputs=+++
  Sum1 : Sum  Inputs=|+-
  Sum2 : Sum  Inputs=++|
  v [m/s] : Outport
  w_w [rad/s] : Outport  Port=2
  wires:
  alpha [rad]/1 -> F0006_gravitationalForce.m/1, F0006_rollingResistance.m/2
  Initial speed/1 -> Integrator2/2
  F0006_airDrag.m/1 -> Sum/1
  F0006_rollingResistance.m/1 -> Sum/2
  Sum1/1 -> Gain/1
  F0006_gravitationalForce.m/1 -> Sum/3
  Gain/1 -> Integrator2/1
  Sum2/1 -> Sum1/2
  Sum/1 -> Sum2/2
  Integrator2/1 -> Divide1/1, Abs1/1, Abs/1, v [m/s]/1
  Abs/1 -> F0006_airDrag.m/1
  Abs1/1 -> F0006_rollingResistance.m/1
  Divide1/1 -> w_w [rad/s]/1
  brake [-]/1 -> F0006_brakeForce.m/1
  F0006_brakeForce.m/1 -> Sum2/1
  Divide/1 -> Sum1/1
  Tq_in [Nm]/1 -> Divide/1
  Constant/1 -> Divide/2, Divide1/2

== system component_lib/Powertrain/PT0002_simpleMotor ==
  Tq_ref [Nm] : Inport
  V [V] : Inport  Port=2
  w_em [rad/s] : Inport  Port=3
  F0009_currentDemand.m : base_lib/F0009_simpleTractionMotor/F0009_currentDemand.m  SystemSampleTime=-1  VariantActivationTime=update diagram  Latency=0  AutoFrameSizeCalculation=off
  Torque dynamics : TransferFcn  Denominator=[T_s 1]
  Tq_em [Nm] : Outport
  I_em [A] : Outport  Port=2
  Q_gen [J/s] : Outport  Port=3
  wires:
  w_em [rad/s]/1 -> F0009_currentDemand.m/3
  V [V]/1 -> F0009_currentDemand.m/2
  Torque dynamics/1 -> Tq_em [Nm]/1, F0009_currentDemand.m/1
  Tq_ref [Nm]/1 -> Torque dynamics/1
  F0009_currentDemand.m/2 -> I_em [A]/1
  F0009_currentDemand.m/1 -> Q_gen [J/s]/1

== system component_lib/Powertrain/PT0003_gearBox ==
  Tq_in [Nm] : Inport
  w_out [rad/s] : Inport  Port=2
  gear  [-] : Inport  Port=3
  clutch  [-] : Inport  Port=4
  1-D Lookup Table : Lookup_n-D  NumberOfTableDimensions=1  BreakpointsForDimension1=par.gears  Table=par.gear_ratios  InterpMethod=Nearest  InternalRulePriority=Speed  RndMeth=Simplest
  F0006_gearBox.m : base_lib/F0006_truckBenchmark/F0006_gearBox.m  SystemSampleTime=-1  VariantActivationTime=update diagram  Latency=0  AutoFrameSizeCalculation=off
  Product : Product
  Tq_out [Nm] : Outport
  w_in [rad/s] : Outport  Port=2
  wires:
  w_out [rad/s]/1 -> F0006_gearBox.m/2
  Tq_in [Nm]/1 -> F0006_gearBox.m/1
  F0006_gearBox.m/2 -> w_in [rad/s]/1
  1-D Lookup Table/1 -> F0006_gearBox.m/3
  gear  [-]/1 -> 1-D Lookup Table/1
  clutch  [-]/1 -> Product/1
  F0006_gearBox.m/1 -> Product/2
  Product/1 -> Tq_out [Nm]/1

== system component_lib/Powertrain/PT0004_electricMachine ==
  I [A] : Inport
  V [V] : Inport  Port=2
  w [rad/s] : Inport  Port=3
  Abs : Abs  SaturateOnIntegerOverflow=off
  Abs1 : Abs  SaturateOnIntegerOverflow=off
  Abs2 : Abs  SaturateOnIntegerOverflow=off
  Constant1 : Constant  Value=V_nom
  Divide : Product  Inputs=**/
  F0009_torque.m : base_lib/F0009_simpleTractionMotor/F0009_torque.m  SystemSampleTime=-1  VariantActivationTime=update diagram  Latency=0  AutoFrameSizeCalculation=off
      settings: LibrarySourceBlock=|
      | simulink/User-Defined
      | Functions/MATLAB Function
  Gain : Gain  Gain=-1
  Product : Product
  Product1 : Product
  Sum : Sum  Inputs=|+-
  Torque Limiter : simulink/Discontinuities/Saturation Dynamic  OutMin=[]  OutMax=[]  OutDataTypeStr=Inherit: Same as second input  OutDataType=fixdt(1, 16)  OutScaling=2^-10  DoSatur=off
  "[0, V_nom]" : Saturate  UpperLimit=V_nom  LowerLimit=0
  "[0,476]" : Saturate  UpperLimit=476  LowerLimit=0
  speed-Torque map1 : Lookup_n-D  NumberOfTableDimensions=1  BreakpointsForDimension1=|  Table=|  ExtrapMethod=Clip  UseLastTableValue=on  InternalRulePriority=Speed  RndMeth=Simplest
      BreakpointsForDimension1=|
      | [25.2590673575129
      | 34.9740932642487
      | 43.3937823834197
      | 51.1658031088083
      | 55.6994818652850
      | 64.1191709844560
      | 65.4145077720207
      | 67.3575129533679
      | 68.0051813471503
      | 69.9481865284974
      | 71.2435233160622
      | 73.1865284974093
      | 75.7772020725389
      | 76.4248704663213
      | 78.3678756476684
      | 81.6062176165803
      | 82.9015544041451
      | 86.1398963730570
      | 88.0829015544041
      | 90.0259067357513
      | 94.5595854922280
      | 97.1502590673575
      | 100.388601036269
      | 103.626943005181
      | 109.455958549223
      | 113.989637305699
      | 120.466321243523
      | 125.000000000000
      | 128.238341968912
      | 133.419689119171
      | 139.248704663212
      | 145.077720207254
      | 150.259067357513
      | 158.031088082902
      | 164.507772020725
      | 172.279792746114
      | 174.870466321244
      | 195.595854922280
      | 211.139896373057
      | 221.502590673575
      | 229.922279792746
      | 244.818652849741
      | 256.476683937824
      | 270.725388601036
      | 284.974093264249
      | 290.155440414508
      | 300.518134715026
      | 313.471502590674
      | 324.481865284974
      | 344.559585492228
      | 356.217616580311
      | 366.580310880829
      | 376.295336787565
      | 384.067357512953
      | 403.497409326425
      | 422.927461139896
      | 438.471502590674
      | 453.367875647669
      | 465.025906735751
      | 476.036269430052]
      Table=|
      | [1991.26637554585
      | 1997.08879184862
      | 1994.17758369723
      | 1994.17758369723
      | 1994.17758369723
      | 1991.26637554585
      | 1944.68704512373
      | 1921.39737991266
      | 1854.43959243086
      | 1816.59388646288
      | 1787.48180494905
      | 1700.14556040757
      | 1671.03347889374
      | 1621.54294032023
      | 1548.76273653566
      | 1513.82823871907
      | 1438.13682678311
      | 1391.55749636099
      | 1339.15574963610
      | 1280.93158660844
      | 1225.61863173217
      | 1176.12809315866
      | 1129.54876273654
      | 1085.88064046579
      | 1018.92285298399
      | 969.432314410480
      | 925.764192139738
      | 876.273653566230
      | 835.516739446870
      | 797.671033478894
      | 756.914119359534
      | 727.802037845706
      | 704.512372634643
      | 666.666666666667
      | 628.820960698690
      | 602.620087336244
      | 588.064046579330
      | 518.195050946142
      | 477.438136826783
      | 445.414847161572
      | 410.480349344978
      | 395.924308588064
      | 375.545851528384
      | 343.522561863173
      | 328.966521106259
      | 320.232896652110
      | 302.765647743814
      | 282.387190684134
      | 282.387190684134
      | 259.097525473071
      | 244.541484716157
      | 244.541484716157
      | 221.251819505094
      | 221.251819505094
      | 209.606986899563
      | 195.050946142649
      | 189.228529839883
      | 183.406113537118
      | 174.672489082969
      | 157.205240174672]
  Tq_em [Nm] : Outport
  Q_gen [J/s] : Outport  Port=2
  wires:
  w [rad/s]/1 -> [w], F0009_torque.m/3
  V [V]/1 -> "[0, V_nom]"/1, F0009_torque.m/1, [V]
  I [A]/1 -> F0009_torque.m/2, [I]
  Divide/1 -> "[0,476]"/1
  "[0,476]"/1 -> speed-Torque map1/1
  Constant1/1 -> Divide/2
  [w] -> Divide/1
  "[0, V_nom]"/1 -> Divide/3
  F0009_torque.m/1 -> Torque Limiter/2
  speed-Torque map1/1 -> Gain/1, Torque Limiter/1
  Torque Limiter/1 -> Product/1, Tq_em [Nm]/1
  Gain/1 -> Torque Limiter/3
  [w] -> Product/2
  [V] -> Product1/1
  [I] -> Product1/2
  Product/1 -> Abs1/1
  Product1/1 -> Abs2/1
  Sum/1 -> Abs/1
  Abs/1 -> Q_gen [J/s]/1
  Abs1/1 -> Sum/1
  Abs2/1 -> Sum/2

== system component_lib/Simple Fuel Cell System/Subsystem1 ==
  note: Rolling Fuel Consumption Calculation [kg/100km]
  In1 : Inport
  Add1 : Sum
  Constant6 : Constant
  Constant7 : Constant  Value=100e3
  Demux : Demux
  Divide : Product  Inputs=**/
  Gain1 : Gain  Gain=-1
  Integrator : Integrator
  SC0002_signalRead11 : $bdroot/Data & Control/SC0002_signalRead  SigName=fuelConsumption
  SC0002_signalRead5 : $bdroot/Data & Control/SC0002_signalRead  SigName=hydrogenFlow
  SC0003_signalWrite1 : $bdroot/Data & Control/SC0003_signalWrite  SigName=distance
  Terminator : Terminator
  Terminator1 : Terminator
  Terminator2 : Terminator
  wires:
  Integrator/1 -> Divide/1
  Constant7/1 -> Divide/2
  SC0003_signalWrite1/1 -> Add1/1
  Demux/1 -> Gain1/1
  Add1/1 -> Divide/3
  Constant6/1 -> Add1/2
  Divide/1 -> SC0002_signalRead11/1
  Gain1/1 -> SC0002_signalRead5/1, Integrator/1
  In1/1 -> Demux/1
  Demux/3 -> Terminator1/1
  Demux/4 -> Terminator2/1
  Demux/2 -> Terminator/1

== system component_lib/Simple Fuel Cell System ITPEM/Subsystem1 ==
  note: Rolling Fuel Consumption Calculation [kg/100km]
  In1 : Inport
  Add1 : Sum
  Constant6 : Constant
  Constant7 : Constant  Value=100e3
  Demux : Demux
  Divide : Product  Inputs=**/
  Gain1 : Gain  Gain=-1
  Integrator : Integrator
  SC0002_signalRead11 : $bdroot/Data & Control/SC0002_signalRead  SigName=fuelConsumption
  SC0002_signalRead5 : $bdroot/Data & Control/SC0002_signalRead  SigName=hydrogenFlow
  SC0003_signalWrite1 : $bdroot/Data & Control/SC0003_signalWrite  SigName=distance
  Terminator : Terminator
  Terminator1 : Terminator
  Terminator2 : Terminator
  wires:
  Integrator/1 -> Divide/1
  Constant7/1 -> Divide/2
  SC0003_signalWrite1/1 -> Add1/1
  Demux/1 -> Gain1/1
  Add1/1 -> Divide/3
  Constant6/1 -> Add1/2
  Divide/1 -> SC0002_signalRead11/1
  Gain1/1 -> SC0002_signalRead5/1, Integrator/1
  In1/1 -> Demux/1
  Demux/3 -> Terminator1/1
  Demux/4 -> Terminator2/1
  Demux/2 -> Terminator/1
